simulink model "active_cell_blancing"  (R2025b)
settings: Solver=ode23s  StartTime=0.0  StopTime=10  RelTol=1e-3
undefined symbols (not defined in the file): Ion, Lithium
libraries: spsIdealSwitchLib x4, spsSeriesRLCBranchLib x4, spsBatteryLib x2, spsDiodeLib x2, spsDCVoltageSourceLib x1, eePwmGeneratorMultilevel x1, spsVoltageMeasurementLib x1, sps_lib x1
settings Model: Creator=hp  LastModifiedBy=hp

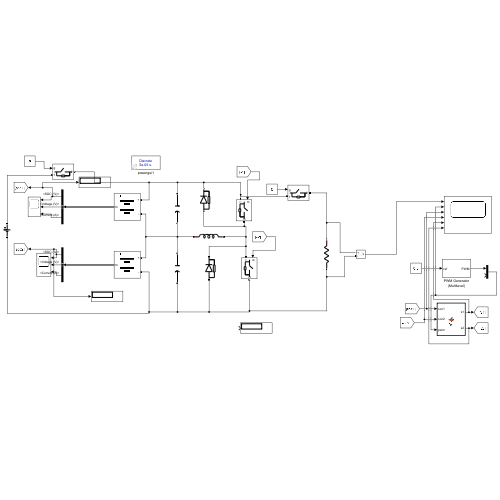
[thumbnail: Simulink's stored preview of the top-level diagram]
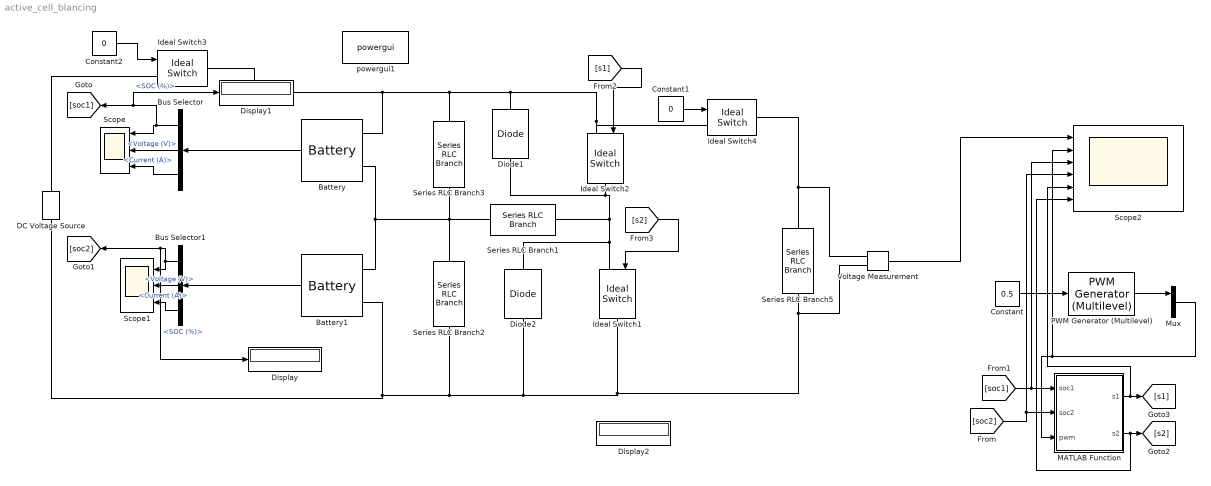
== system active_cell_blancing ==
  Battery : spsBatteryLib/Battery  BatType=Lithium-Ion  NomV=3.2  NomQ=6  SOC=50  Batt_Tr=1  PresetModel=off  MaxQ=6  MinV=2.5  FullV=3.65  Dis_rate=2  R=0.0053333  Normal_OP=5.4261  expZone="[3.4572     0.29478]"
  Battery1 : spsBatteryLib/Battery  BatType=Lithium-Ion  NomV=3.2  NomQ=6  SOC=35  Batt_Tr=1  PresetModel=off  MaxQ=6  MinV=2.5  FullV=3.65  Dis_rate=2  R=0.0053333  Normal_OP=5.4261  expZone="[3.4572     0.29478]"
  Bus Selector : BusSelector  OutputSignals=SOC (%),Voltage (V),Current (A)
  Bus Selector1 : BusSelector  OutputSignals=SOC (%),Voltage (V),Current (A)
  Constant : Constant  Value=0.5
  Constant1 : Constant  Value=0
  Constant2 : Constant  Value=0
  DC Voltage Source : spsDCVoltageSourceLib/DC Voltage Source  Amplitude=12  Measurements=None
  Diode1 : spsDiodeLib/Diode  Ron=0.001  Lon=0  Vf=0.8  IC=0  UseSnubber=off  Rs=50000  Cs=250e-9  Measurements=off
  Diode2 : spsDiodeLib/Diode  Ron=0.001  Lon=0  Vf=0.8  IC=0  UseSnubber=off  Rs=50000  Cs=250e-9  Measurements=off
  Display : Display
  Display1 : Display
  Display2 : Display
  Ideal Switch{1..4} (4 alike) : spsIdealSwitchLib/Ideal Switch  Ron=0.001  Lon=0  IC=0  Rs=1e5  Cs=inf  Measurements=off
  MATLAB Function : MATLAB Function  TreatAsAtomicUnit=on
  Mux : Mux  Inputs=2
  PWM Generator (Multilevel) : eePwmGeneratorMultilevel/PWM Generator (Multilevel)  topology=Half-bridge  Nsm=2  Tper=1/10000  Ts=0
      settings: LibrarySourceBlock=|
      | ee_sl_lib/Pulse Width
      | Modulation/PWM Generator
      | (Multilevel)
  Scope : Scope  NumInputPorts=3
      settings: ActiveDisplayYMinimum=-1  ActiveDisplayYMaximum=1
  Scope1 : Scope  NumInputPorts=3
  Scope2 : Scope  NumInputPorts=6
      settings: ActiveDisplayYMinimum=-1  ActiveDisplayYMaximum=1  DataLoggingVariableName=ScopeData2
  Series RLC Branch1 : spsSeriesRLCBranchLib/Series RLC Branch  LConnTagsString=__new0  RConnTagsString=__new0  BranchType=L  Resistance=50  Inductance=1e-3  SetiL0=off  InitialCurrent=0  Capacitance=1e-6  Setx0=off  InitialVoltage=0  Measurements=None
  Series RLC Branch2 : spsSeriesRLCBranchLib/Series RLC Branch  LConnTagsString=__new0  RConnTagsString=__new0  BranchType=C  Resistance=50  Inductance=3e-3  SetiL0=off  InitialCurrent=0  Capacitance=1e-6  Setx0=off  InitialVoltage=0  Measurements=None
  Series RLC Branch3 : spsSeriesRLCBranchLib/Series RLC Branch  LConnTagsString=__new0  RConnTagsString=__new0  BranchType=C  Resistance=50  Inductance=3e-3  SetiL0=off  InitialCurrent=0  Capacitance=1e-6  Setx0=off  InitialVoltage=0  Measurements=None
  Series RLC Branch5 : spsSeriesRLCBranchLib/Series RLC Branch  LConnTagsString=__new0  RConnTagsString=__new0  BranchType=R  Resistance=10  Inductance=1e-3  SetiL0=off  InitialCurrent=0  Capacitance=1e-6  Setx0=off  InitialVoltage=0  Measurements=None
  Voltage Measurement : spsVoltageMeasurementLib/Voltage Measurement  PhasorSimulation=off  OutputType=Complex  PSBequivalent=0
  powergui1 : sps_lib/powergui  Priority=1  SimulationMode=Discrete  SampleTime=50e-6  frequency=60  Iterations=50  frequencyindice=0  Pbase=100e6  ErrMax=1e-4  UnitsV=kV  UnitsW=MW  buscounter=0  FunctionMessages=off  echomessages=off  EnableUseOfTLC=off  CurrentSourceSwitches=off  DisableSnubberDevices=off  DisableRonSwitches=off  DisableVfSwitches=off  DisplayEquations=off  AutomaticDiscreteSolvers=off  SolverType=Tustin/Backward Euler (TBE)  Interpol=off  ExternalGateDelay=off  methode=off  Ts=100  x0status=blocks  SPID=on  SwTol=0  HookPort=off  NonlinearTolerance=1e-4  nMaxIteration=100  ContinueOnMaxIteration=off  RestoreLinks=warning  ResistiveCurrentMeasurement=off  Frange=[0:2:500]  Ylog=off  Xlog=on  ShowGrid=off  save=off  variable=ZData  structure=0  ZoomFFT=off  StartTime=0.0  cycles=1  DisplayStyle=1  fundamental=60  FreqAxis=off  MaxFrequency=1000  frequencyindicesteady=1  RmsSteady=1  display=off
  wires:
  Battery/1 -> Bus Selector/1
  Battery1/1 -> Bus Selector1/1
  Constant/1 -> PWM Generator (Multilevel)/1
  PWM Generator (Multilevel)/1 -> Mux/1
  Bus Selector/2 -> Scope/2  "<Voltage (V)>"
  Bus Selector/1 -> Display1/1, [soc1], Scope/1  "<SOC (%)>"
  Bus Selector/3 -> Scope/3  "<Current (A)>"
  Bus Selector1/1 -> Scope1/1, [soc2], Display/1  "<SOC (%)>"
  Bus Selector1/2 -> Scope1/2  "<Voltage (V)>"
  Bus Selector1/3 -> Scope1/3  "<Current (A)>"
  [soc1] -> Scope2/3, MATLAB Function/1(soc1)
  [soc2] -> Scope2/4, MATLAB Function/2(soc2)
  Mux/1 -> Scope2/2, MATLAB Function/3(pwm)
  MATLAB Function/1(s1) -> Scope2/5, [s1]
  MATLAB Function/2(s2) -> Scope2/6, [s2]
  [s1] -> Ideal Switch2/1
  [s2] -> Ideal Switch1/1
  Voltage Measurement/1 -> Scope2/1
  Constant1/1 -> Ideal Switch4/1
  Constant2/1 -> Ideal Switch3/1
  connections:
  DC Voltage Source/LConn1 -- Series RLC Branch5/RConn1 -- Voltage Measurement/LConn2 -- Ideal Switch1/RConn1 -- Diode2/LConn1 -- Series RLC Branch2/RConn1 -- Battery1/LConn2
  Diode1/LConn1 -- Diode2/RConn1 -- Ideal Switch1/LConn1 -- Series RLC Branch1/RConn1 -- Ideal Switch2/RConn1
  Ideal Switch3/LConn1 -- DC Voltage Source/RConn1
  Ideal Switch2/LConn1 -- Diode1/RConn1 -- Series RLC Branch3/LConn1 -- Battery/LConn1 -- Ideal Switch3/RConn1 -- Ideal Switch4/LConn1
  Ideal Switch4/RConn1 -- Series RLC Branch5/LConn1 -- Voltage Measurement/LConn1
  Battery/LConn2 -- Series RLC Branch1/LConn1 -- Series RLC Branch3/RConn1 -- Series RLC Branch2/LConn1 -- Battery1/LConn1

== matlab function active_cell_blancing/MATLAB Function ==
  data: soc1 input; s1 output; soc2 input; pwm input; s2 output
function [s1 , s2] = fcn(soc1,soc2,pwm)
p=pwm(1);
if soc2 < soc1
    s1=p
    s2=0
elseif soc1 < soc2
    s1 =0
    s2 =p
else
    s1=0
    s2=0

end
